simulink model "S_matrix"  (Simulink 8.0)
settings: Solver=ode45  StartTime=0.0  StopTime=10.0  RelTol=1e-3
undefined symbols (not defined in the file or in its folder): i
settings Model: Creator=Faradars  LastModifiedBy=Faradars

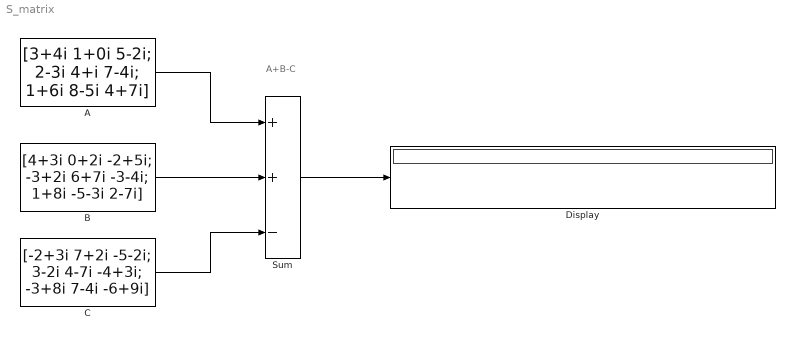
== system S_matrix ==
  note: A+B-C
  A : Constant  Value=[3+4i 1+0i 5-2i; 2-3i 4+i 7-4i; 1+6i 8-5i 4+7i]
  B : Constant  Value=[4+3i 0+2i -2+5i; -3+2i 6+7i -3-4i; 1+8i -5-3i 2-7i]
  C : Constant  Value=[-2+3i 7+2i -5-2i; 3-2i 4-7i -4+3i; -3+8i 7-4i -6+9i]
  Display : Display
  Sum : Sum  Inputs=++-
  wires:
  Sum/1 -> Display/1
  A/1 -> Sum/1
  B/1 -> Sum/2
  C/1 -> Sum/3
